simulink model "noise_block_test"  (R2015a)
settings: Solver=ode45  StartTime=0.0  StopTime=Tsim  MaxStep=Tsim/10000  RelTol=1e-3
libraries: dspstat3 x1
settings Model: Creator=mainster  LastModifiedBy=mainster

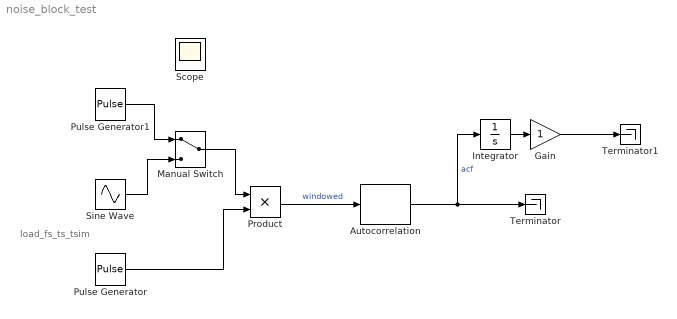
== system noise_block_test ==
  note: load_fs_ts_tsim
  Autocorrelation : dspstat3/Autocorrelation  AllPositiveLags=on  maxlag=1  bias=None  domain=Time  outputDataTypeStr=Inherit: Same as accumulator  outputLastDataTypeStr=Inherit: Same as accumulator  outputMin=[]  outputMax=[]  roundingMode=Floor  overflowMode=off
  Gain : Gain
  Integrator : Integrator
  Manual Switch : ManualSwitch
  Product : Product
  Pulse Generator : DiscretePulseGenerator  PulseType=Time based  Period=100  PulseWidth=80  PhaseDelay=10
  Pulse Generator1 : DiscretePulseGenerator  PulseType=Time based  Period=2*pi  PulseWidth=50
  Sine Wave : Sin
  Terminator : Terminator
  Terminator1 : Terminator
  Scope : Scope  NumInputPorts=3
      settings: ShowLegends=on  TimeRange=100  YMin=-1~-5~-5  YMax=1~5~5  ScrollMode=on
  wires:
  Autocorrelation/1 -> Integrator/1, Terminator/1  "acf"
  Sine Wave/1 -> Manual Switch/2
  Integrator/1 -> Gain/1
  Gain/1 -> Terminator1/1
  Product/1 -> Autocorrelation/1  "windowed"
  Pulse Generator/1 -> Product/2
  Pulse Generator1/1 -> Manual Switch/1
  Manual Switch/1 -> Product/1
